simulink model "Sistema_in_catena_aperta"  (R2014a)
settings: Solver=ode45  StartTime=0.0  StopTime=20  RelTol=1e-3
values from neighbouring files (symbols this model uses):
  F1 = Ka*Km/(s^2*J*La + s*(beta*La + J*Ra) + beta*Ra + Km^2)    [E02.m]
  F2 = -(s*La + Ra)/(s^2*J*La + s*(beta*La + J*Ra) + beta*Ra + Km^2)    [E02.m]
  s = tf('s')    [E02.m]
libraries: cstblocks x2
settings Model: Creator=Davide  LastModifiedBy=Davide

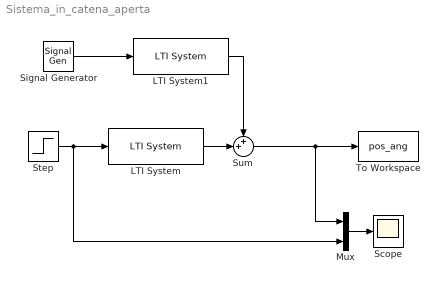
== system Sistema_in_catena_aperta ==
  LTI System : cstblocks/LTI System  sys=F1/s  IC=[]
  LTI System1 : cstblocks/LTI System  sys=F2/s  IC=[]
  Mux : Mux  Inputs=2
  Scope : Scope
  Signal Generator : SignalGenerator  WaveForm=square  Amplitude=0.05  Frequency=0.1
  Step : Step  Time=0  SampleTime=0
  Sum : Sum  Inputs=++|
  To Workspace : ToWorkspace  VariableName=pos_ang  SaveFormat=Timeseries  SampleTime=-1
  wires:
  Step/1 -> Mux/2, LTI System/1
  LTI System/1 -> Sum/2
  LTI System1/1 -> Sum/1
  Signal Generator/1 -> LTI System1/1
  Sum/1 -> To Workspace/1, Mux/1
  Mux/1 -> Scope/1
